simulink model "UUV_sim"  (Simulink 8.3)
settings: Solver=ode45  StartTime=0.0  StopTime=1000  RelTol=1e-3
undefined symbols (not defined in the file): drawUUV, P
libraries: cstblocks x1, simulink x1
settings Model: Creator=beard  LastModifiedBy=jhl48
settings OptimizationCC: ExpressionDepthLimit=2147483647  InitFltsAndDblsToZero=on
settings DebuggingCC: FcnCallInpInsideContextMsg=UseLocalSettings

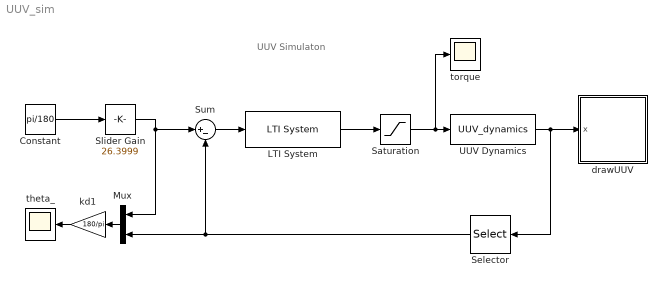
== system UUV_sim ==
  note: UUV Simulaton
  Constant : Constant  Value=pi/180
  LTI System : cstblocks/LTI System  sys=C  IC=[]
  Mux : Mux  Inputs=2
  Saturation : Saturate  UpperLimit=P.tau_max  LowerLimit=-P.tau_max
  Selector : Selector  InputPortWidth=2  Indices=[1]
  Slider Gain : simulink/Math Operations/Slider Gain  low=-180  gain=26.3999  high=180
  Sum : Sum  Inputs=|+-
  UUV Dynamics : S-Function  FunctionName=UUV_dynamics  Parameters=P  EnableBusSupport=off
  drawUUV : Subsystem
      mask init:
      | % drawing parameters
      | MajorAxis = 10;
      | MinorAxis = 6;
      | C_M = [0;-4];
      mask Display: image(imread('tv.jpg'))
  kd1 : Gain  Gain=180/pi
  theta_ : Scope
      settings: YMin=20  YMax=32
  torque : Scope
      settings: YMin=5.55112e-17  YMax=1
  wires:
  UUV Dynamics/1 -> drawUUV/1(x), Selector/1
  Saturation/1 -> UUV Dynamics/1, torque/1
  Mux/1 -> kd1/1
  kd1/1 -> theta_/1
  LTI System/1 -> Saturation/1
  Constant/1 -> Slider Gain/1
  Slider Gain/1 -> Sum/1, Mux/1
  Selector/1 -> Sum/2, Mux/2
  Sum/1 -> LTI System/1

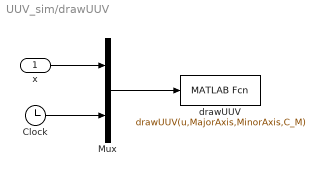
== system UUV_sim/drawUUV ==
  x : Inport
  Clock : Clock
  Mux : Mux  Inputs=2
  drawUUV : MATLABFcn  MATLABFcn=drawUUV(u,MajorAxis,MinorAxis,C_M)  OutputDimensions=0  SampleTime=0.1
  wires:
  Mux/1 -> drawUUV/1
  x/1 -> Mux/1
  Clock/1 -> Mux/2
